simulink model "bb_pid_hg_sl"  (Simulink 8.7)
settings: Solver=FixedStepDiscrete  StartTime=0.0  StopTime=inf  FixedStep=ts  RelTol=1e-3
values from neighbouring files (symbols this model uses):
  K_theta_hg = (pi/180)*(2.1/14.1)    (= 0.00259942654552)    [bb_pid_hg.m]
  Kd = -((p1+p2)*T + 1)/K    [bb_pid_hg.m]
  kd = -(p1+p2+p3)/K_b    [bb_pid_hg.m]
  kff = ki/alpha    [bb_pid_hg.m]
  ki = -p1*p2*p3/K_b    [bb_pid_hg.m]
  Kp = p1*p2*T/K    [bb_pid_hg.m]
  kp = (p1*p2 + p2*p3 + p3*p1)/K_b    [bb_pid_hg.m]
  r1 = 20-5    (= 15)    [bb_pid_hg.m]
  r2 = 20+5    (= 25)    [bb_pid_hg.m]
undefined symbols (not defined in the file or in its folder): denbd, denlpf, denpd, DiscIntNeverNeededParam, numbd, numlpf, numpd, r, r_cyc, ts
libraries: arduinolib x4, simulink x4
settings Model: Creator=hirata  LastModifiedBy=morita  SimulationMode=external  ExtModeTrigDuration=2
settings DataIOCC: SignalLoggingSaveFormat=ModelDataLogs
settings OptimizationCC: ExpressionDepthLimit=2147483647  OptimizeModelRefInitCode=on  LifeSpan=Inf  MaxStackSize=64
settings DebuggingCC: SolverPrmCheckMsg=warning  FcnCallInpInsideContextMsg=UseLocalSettings  StateNameClashWarn=warning
settings HardwareCC: ProdBitPerInt=16  ProdBitPerPointer=16  ProdIntDivRoundTo=Zero  ProdEndianess=LittleEndian  ProdWordSize=8  ProdHWDeviceType=Atmel->AVR  UseEmbeddedCoderFeatures=off  UseSimulinkCoderFeatures=off
settings RTWCC: SystemTargetFile=ert.tlc  HardwareBoard=Arduino Mega 2560  TLCOptions=-aInlineSetEventsForThisBaseRateFcn=TLC_FALSE -aSuppressMultiTaskScheduler=TLC_FALSE  TemplateMakefile=ert_default_tmf  Description=Embedded Coder  GenerateReport=on  Toolchain=Arduino AVR v1.6.1  BuildConfiguration=Faster Runs  IncludeHyperlinkInReport=on  LaunchReport=on  GenerateTraceInfo=on  GenerateTraceReport=on  GenerateTraceReportSl=on  GenerateTraceReportSf=on  GenerateTraceReportEml=on
settings MATStruct: className=codertarget.tools.BuildHook  argsTopModelOnly=[]  excludedModels=[]  includeReferencedModels=on  includeTopModel=on  enabled=on  UseCoderTarget=[1]  TargetHardware=Arduino Mega 2560  RTOS=Baremetal  Scheduler_interrupt_source=[0.0]  DataVersion=2016.02  Baudrate=115200  COMPort=codertarget.arduinobase.internal.getExternalModeMexArgs('Serial')  Verbose=[0]  IPAddress=codertarget.arduinobase.internal.getExternalModeMexArgs('Ethernet')  Port=17725  Configuration=Serial  BuildAction=Build, load and run  Set_host_COM_port=Automatically  COM_port_number=1  Enable_overrun_detection=[0.0]  Digital_output_to_set_on_overrun=13  Analog_input_reference_voltage=[0.0]  Serial0_baud_rate=9600  Serial1_baud_rate=9600  Serial2_baud_rate=9600  Serial3_baud_rate=9600  SPI_clock_out_frequency=4000  SPI_mode=Mode 0 - Clock Polarity 0, Clock Phase 0  SPI_bitorder=MSB first  Disable_DHCP_Ethernet=[0.0]  Local_ip_address=192.168.0.20  Local_mac_address=DE:AD:BE:EF:FE:ED  Disable_DHCP_Wifi=[0.0]  Wifi_ip_address=192.168.1.20  Wifi_SSID=yourNetwork  Set_Wifi_Encryption=None  Wifi_WEP_key=D0D0DEADF00DABBADEAFBEADED  Wifi_WEP_key_index=0  Wifi_WPA_password=secretPassword
settings CodeAppCC: ForceParamTrailComments=on  IgnoreCustomStorageClasses=off  OperatorAnnotations=on  SimulinkDataObjDesc=on  SFDataObjDesc=on  MATLABFcnDesc=on  InsertBlockDesc=on  MATLABSourceComments=on
settings ERTTargetCC: MultiwordLength=2048  SupportContinuousTime=on  SupportNonInlinedSFcns=on  SupportVariableSizeSignals=on

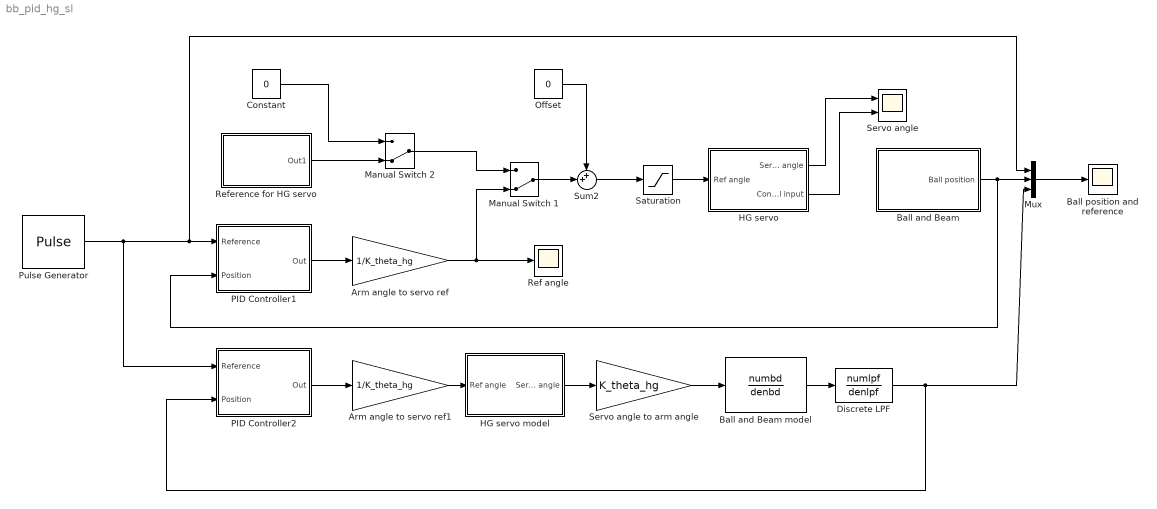
== system bb_pid_hg_sl ==
  Arm angle to servo ref : Gain  Gain=1/K_theta_hg
  Arm angle to servo ref1 : Gain  Gain=1/K_theta_hg
  Ball and Beam : Subsystem
  Ball and Beam model : DiscreteTransferFcn  Numerator=numbd  Denominator=denbd
  Ball position and reference : Scope
  Constant : Constant  Value=0
  Discrete LPF : DiscreteTransferFcn  Numerator=numlpf  Denominator=denlpf
  HG servo : Subsystem
  HG servo model : Subsystem
  Manual Switch 1 : ManualSwitch  CurrentSetting=0
  Manual Switch 2 : ManualSwitch  CurrentSetting=0
  Mux : Mux  Inputs=3
  Offset : Constant  Value=0  SampleTime=ts
  PID Controller1 : Subsystem
  PID Controller2 : Subsystem
  Pulse Generator : DiscretePulseGenerator  PulseType=Time based  Amplitude=r2-r1  Period=30  PulseWidth=50  PhaseDelay=10
  Ref angle : Scope
  Reference for HG servo : Subsystem
  Saturation : Saturate  UpperLimit=45  LowerLimit=-45
  Servo angle : Scope  NumInputPorts=2
  Servo angle to arm angle : Gain  Gain=K_theta_hg
  Sum2 : Sum  Inputs=++|
  wires:
  Offset/1 -> Sum2/1
  Arm angle to servo ref/1 -> Manual Switch 1/2, Ref angle/1
  Sum2/1 -> Saturation/1
  Mux/1 -> Ball position and reference/1
  Manual Switch 1/1 -> Sum2/2
  Saturation/1 -> HG servo/1(Ref angle)
  Ball and Beam/1(Ball position) -> Mux/2, PID Controller1/2(Position)
  Pulse Generator/1 -> Mux/1, PID Controller1/1(Reference), PID Controller2/1(Reference)
  Ball and Beam model/1 -> Discrete LPF/1
  PID Controller1/1(Out) -> Arm angle to servo ref/1
  Discrete LPF/1 -> Mux/3, PID Controller2/2(Position)
  HG servo/1(Servo angle) -> Servo angle/1
  HG servo/2(Control input) -> Servo angle/2
  Arm angle to servo ref1/1 -> HG servo model/1(Ref angle)
  HG servo model/1(Servo angle) -> Servo angle to arm angle/1
  PID Controller2/1(Out) -> Arm angle to servo ref1/1
  Servo angle to arm angle/1 -> Ball and Beam model/1
  Manual Switch 2/1 -> Manual Switch 1/1
  Reference for HG servo/1(Out1) -> Manual Switch 2/2
  Constant/1 -> Manual Switch 2/1

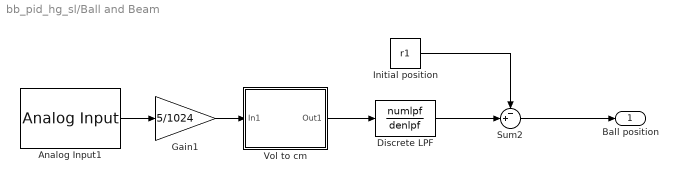
== system bb_pid_hg_sl/Ball and Beam ==
  Analog Input1 : arduinolib/Analog Input  pinNumber=2  sampleTime=ts  blockPlatform=arduino
  Discrete LPF : DiscreteTransferFcn  Numerator=numlpf  Denominator=denlpf
  Gain1 : Gain  Gain=5/1024
  Initial position : Constant  Value=r1
  Sum2 : Sum  Inputs=-+|
  Vol to cm : Subsystem
  Ball position : Outport
  wires:
  Analog Input1/1 -> Gain1/1
  Gain1/1 -> Vol to cm/1(In1)
  Vol to cm/1(Out1) -> Discrete LPF/1
  Initial position/1 -> Sum2/1
  Discrete LPF/1 -> Sum2/2
  Sum2/1 -> Ball position/1

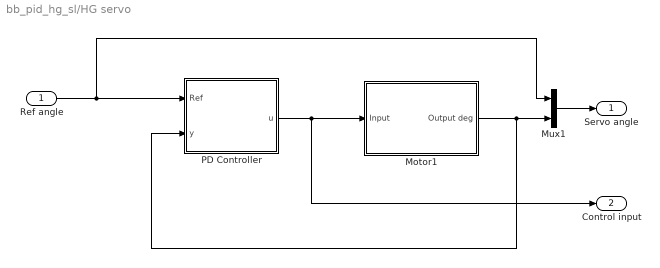
== system bb_pid_hg_sl/HG servo ==
  Ref angle : Inport
  Motor1 : Subsystem
  Mux1 : Mux  Inputs=2
  PD Controller : Subsystem
  Servo angle : Outport
  Control input : Outport  Port=2
  wires:
  Mux1/1 -> Servo angle/1
  Motor1/1(Output deg) -> Mux1/2, PD Controller/2(y)
  Ref angle/1 -> Mux1/1, PD Controller/1(Ref)
  PD Controller/1(u) -> Motor1/1(Input), Control input/1

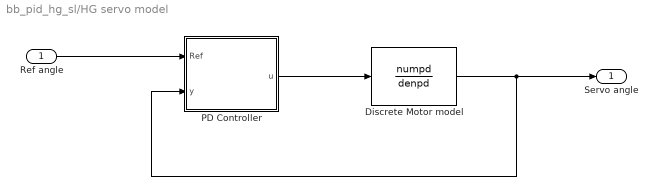
== system bb_pid_hg_sl/HG servo model ==
  Ref angle : Inport
  Discrete Motor model : DiscreteTransferFcn  Numerator=numpd  Denominator=denpd
  PD Controller : Subsystem
  Servo angle : Outport
  wires:
  Ref angle/1 -> PD Controller/1(Ref)
  PD Controller/1(u) -> Discrete Motor model/1
  Discrete Motor model/1 -> Servo angle/1, PD Controller/2(y)

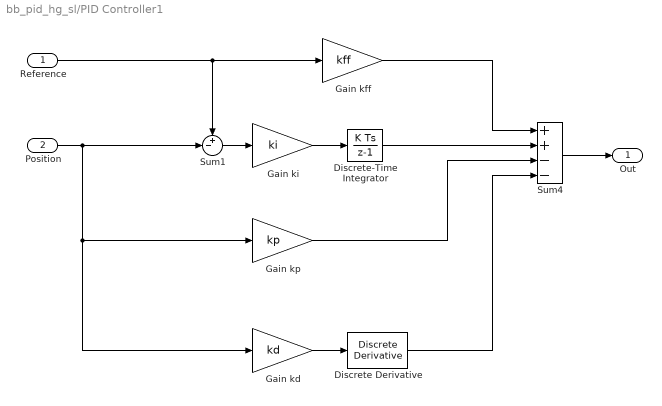
== system bb_pid_hg_sl/PID Controller1 ==
  Reference : Inport
  Position : Inport  Port=2
  Discrete Derivative : simulink/Discrete/Discrete Derivative  gainval=1.0  ICPrevScaledInput=0.0  InputProcessing=Inherited  OutMin=[]  OutMax=[]  OutDataType=fixdt(1, 16)  OutScaling=2^-10  DoSatur=off
  Discrete-Time Integrator : DiscreteIntegrator  SampleTime=ts  ICPrevOutput=DiscIntNeverNeededParam  ICPrevScaledInput=DiscIntNeverNeededParam
  Gain kd : Gain  Gain=kd
  Gain kff : Gain  Gain=kff
  Gain ki : Gain  Gain=ki
  Gain kp : Gain  Gain=kp
  Sum1 : Sum  Inputs=+-|
  Sum4 : Sum  Inputs=++--
  Out : Outport
  wires:
  Reference/1 -> Sum1/1, Gain kff/1
  Sum1/1 -> Gain ki/1
  Position/1 -> Sum1/2, Gain kp/1, Gain kd/1
  Discrete-Time Integrator/1 -> Sum4/2
  Gain ki/1 -> Discrete-Time Integrator/1
  Sum4/1 -> Out/1
  Gain kff/1 -> Sum4/1
  Gain kp/1 -> Sum4/3
  Gain kd/1 -> Discrete Derivative/1
  Discrete Derivative/1 -> Sum4/4

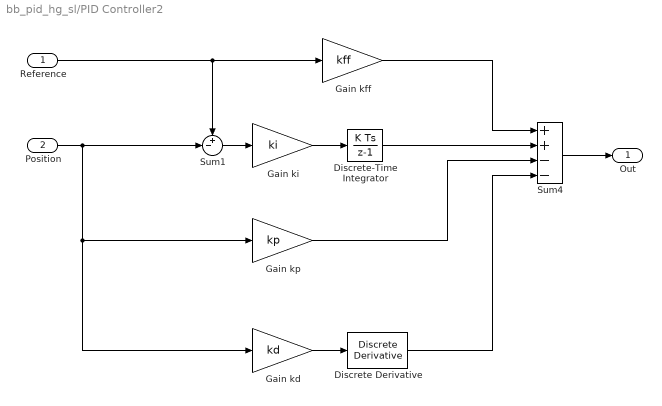
== system bb_pid_hg_sl/PID Controller2 ==
  Reference : Inport
  Position : Inport  Port=2
  Discrete Derivative : simulink/Discrete/Discrete Derivative  gainval=1.0  ICPrevScaledInput=0.0  InputProcessing=Inherited  OutMin=[]  OutMax=[]  OutDataType=fixdt(1, 16)  OutScaling=2^-10  DoSatur=off
  Discrete-Time Integrator : DiscreteIntegrator  SampleTime=ts  ICPrevOutput=DiscIntNeverNeededParam  ICPrevScaledInput=DiscIntNeverNeededParam
  Gain kd : Gain  Gain=kd
  Gain kff : Gain  Gain=kff
  Gain ki : Gain  Gain=ki
  Gain kp : Gain  Gain=kp
  Sum1 : Sum  Inputs=+-|
  Sum4 : Sum  Inputs=++--
  Out : Outport
  wires:
  Reference/1 -> Sum1/1, Gain kff/1
  Sum1/1 -> Gain ki/1
  Position/1 -> Sum1/2, Gain kp/1, Gain kd/1
  Discrete-Time Integrator/1 -> Sum4/2
  Gain ki/1 -> Discrete-Time Integrator/1
  Sum4/1 -> Out/1
  Gain kff/1 -> Sum4/1
  Gain kp/1 -> Sum4/3
  Gain kd/1 -> Discrete Derivative/1
  Discrete Derivative/1 -> Sum4/4

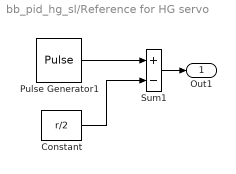
== system bb_pid_hg_sl/Reference for HG servo ==
  Constant : Constant  Value=r/2
  Pulse Generator1 : DiscretePulseGenerator  PulseType=Time based  Amplitude=r  Period=r_cyc  PulseWidth=50
  Sum1 : Sum  Inputs=+-
  Out1 : Outport
  wires:
  Pulse Generator1/1 -> Sum1/1
  Constant/1 -> Sum1/2
  Sum1/1 -> Out1/1

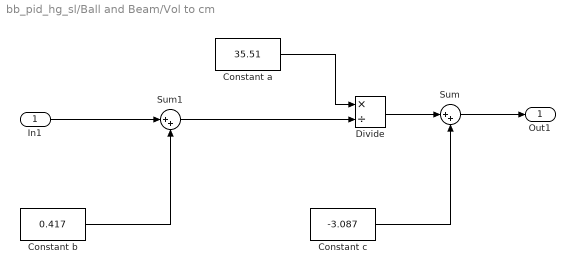
== system bb_pid_hg_sl/Ball and Beam/Vol to cm ==
  In1 : Inport
  Constant a : Constant  Value=35.51
  Constant b : Constant  Value=0.417
  Constant c : Constant  Value=-3.087
  Divide : Product  Inputs=*/
  Sum : Sum  Inputs=|++
  Sum1 : Sum  Inputs=|++
  Out1 : Outport
  wires:
  Constant a/1 -> Divide/1
  Divide/1 -> Sum/1
  Sum/1 -> Out1/1
  Constant c/1 -> Sum/2
  In1/1 -> Sum1/1
  Sum1/1 -> Divide/2
  Constant b/1 -> Sum1/2

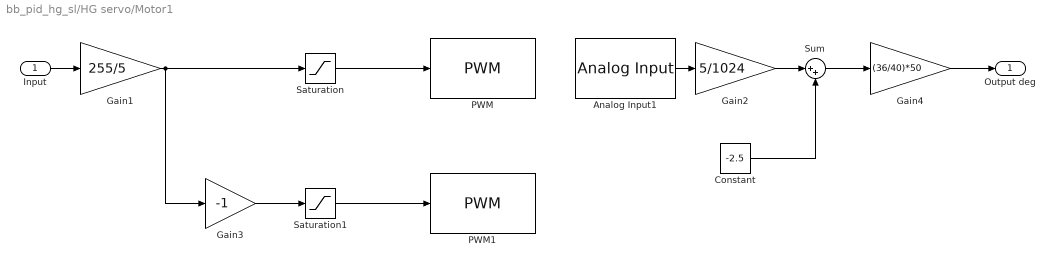
== system bb_pid_hg_sl/HG servo/Motor1 ==
  Input : Inport
  Analog Input1 : arduinolib/Analog Input  pinNumber=0  sampleTime=ts  blockPlatform=arduino
  Constant : Constant  Value=-2.5
  Gain1 : Gain  Gain=255/5
  Gain2 : Gain  Gain=5/1024
  Gain3 : Gain  Gain=-1
  Gain4 : Gain  Gain=(36/40)*50
  PWM : arduinolib/PWM  pinNumber=3  blockPlatform=arduino
  PWM1 : arduinolib/PWM  pinNumber=5  blockPlatform=arduino
  Saturation : Saturate  UpperLimit=255  LowerLimit=0
  Saturation1 : Saturate  UpperLimit=255  LowerLimit=0
  Sum : Sum  Inputs=|++
  Output deg : Outport
  wires:
  Input/1 -> Gain1/1
  Analog Input1/1 -> Gain2/1
  Saturation/1 -> PWM/1
  Gain1/1 -> Gain3/1, Saturation/1
  Saturation1/1 -> PWM1/1
  Gain4/1 -> Output deg/1
  Gain2/1 -> Sum/1
  Sum/1 -> Gain4/1
  Constant/1 -> Sum/2
  Gain3/1 -> Saturation1/1

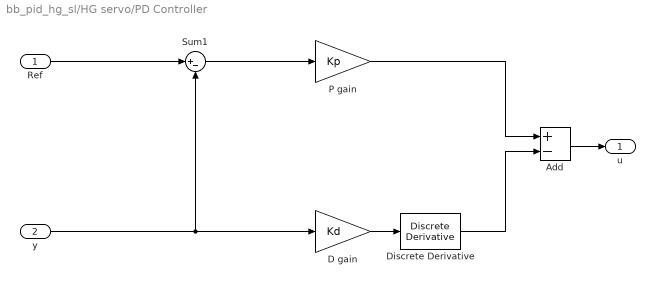
== system bb_pid_hg_sl/HG servo/PD Controller ==
  Ref : Inport
  y : Inport  Port=2
  Add : Sum  Inputs=+-
  D gain : Gain  Gain=Kd
  Discrete Derivative : simulink/Discrete/Discrete Derivative  gainval=1.0  ICPrevScaledInput=0.0  InputProcessing=Inherited  OutMin=[]  OutMax=[]  OutDataType=fixdt(1, 16)  OutScaling=2^-10  DoSatur=off
  P gain : Gain  Gain=Kp
  Sum1 : Sum  Inputs=|+-
  u : Outport
  wires:
  D gain/1 -> Discrete Derivative/1
  Discrete Derivative/1 -> Add/2
  Add/1 -> u/1
  Ref/1 -> Sum1/1
  P gain/1 -> Add/1
  y/1 -> D gain/1, Sum1/2
  Sum1/1 -> P gain/1

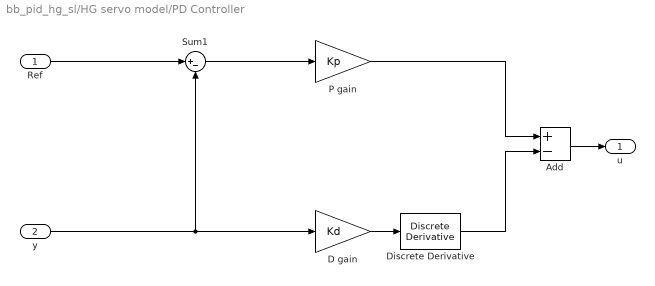
== system bb_pid_hg_sl/HG servo model/PD Controller ==
  Ref : Inport
  y : Inport  Port=2
  Add : Sum  Inputs=+-
  D gain : Gain  Gain=Kd
  Discrete Derivative : simulink/Discrete/Discrete Derivative  gainval=1.0  ICPrevScaledInput=0.0  InputProcessing=Inherited  OutMin=[]  OutMax=[]  OutDataType=fixdt(1, 16)  OutScaling=2^-10  DoSatur=off
  P gain : Gain  Gain=Kp
  Sum1 : Sum  Inputs=|+-
  u : Outport
  wires:
  Sum1/1 -> P gain/1
  y/1 -> Sum1/2, D gain/1
  P gain/1 -> Add/1
  Ref/1 -> Sum1/1
  Add/1 -> u/1
  Discrete Derivative/1 -> Add/2
  D gain/1 -> Discrete Derivative/1
